simulink model "Block Diagram"  (R2024b)
settings: Solver=VariableStepAuto  StartTime=0.0  StopTime=10.0  RelTol=1e-3
libraries: simulink_extras x43, eeGeneralControl x4
(part 3 of 3)

== system Block Diagram/ALU/9-bit RCA/9bitRCA/1bitFAC2 ==
  y : Inport
  x : Inport  Port=2
  cin : Inport  Port=3
  AND : Logic  IconShape=distinctive  AllPortsSameDT=off  OutDataTypeStr=boolean
  AND1 : Logic  IconShape=distinctive  AllPortsSameDT=off  OutDataTypeStr=boolean
  AND2 : Logic  IconShape=distinctive  AllPortsSameDT=off  OutDataTypeStr=boolean
  OR : Logic  Operator=OR  Inputs=3  IconShape=distinctive  AllPortsSameDT=off  OutDataTypeStr=boolean
  XOR : Logic  Operator=XOR  Inputs=3  IconShape=distinctive  AllPortsSameDT=off  OutDataTypeStr=boolean
  z : Outport
  cout : Outport  Port=2
  wires:
  y/1 -> AND2/1, AND/2, XOR/2
  x/1 -> AND1/1, AND/1, XOR/1
  cin/1 -> AND2/2, AND1/2, XOR/3
  XOR/1 -> z/1
  OR/1 -> cout/1
  AND/1 -> OR/1
  AND1/1 -> OR/2
  AND2/1 -> OR/3

== system Block Diagram/ALU/9-bit RCA/9bitRCA/1bitFAC3 ==
  y : Inport
  x : Inport  Port=2
  cin : Inport  Port=3
  AND : Logic  IconShape=distinctive  AllPortsSameDT=off  OutDataTypeStr=boolean
  AND1 : Logic  IconShape=distinctive  AllPortsSameDT=off  OutDataTypeStr=boolean
  AND2 : Logic  IconShape=distinctive  AllPortsSameDT=off  OutDataTypeStr=boolean
  OR : Logic  Operator=OR  Inputs=3  IconShape=distinctive  AllPortsSameDT=off  OutDataTypeStr=boolean
  XOR : Logic  Operator=XOR  Inputs=3  IconShape=distinctive  AllPortsSameDT=off  OutDataTypeStr=boolean
  z : Outport
  cout : Outport  Port=2
  wires:
  y/1 -> AND2/1, AND/2, XOR/2
  x/1 -> AND1/1, AND/1, XOR/1
  cin/1 -> AND2/2, AND1/2, XOR/3
  XOR/1 -> z/1
  OR/1 -> cout/1
  AND/1 -> OR/1
  AND1/1 -> OR/2
  AND2/1 -> OR/3

== system Block Diagram/ALU/9-bit RCA/9bitRCA/1bitFAC4 ==
  y : Inport
  x : Inport  Port=2
  cin : Inport  Port=3
  AND : Logic  IconShape=distinctive  AllPortsSameDT=off  OutDataTypeStr=boolean
  AND1 : Logic  IconShape=distinctive  AllPortsSameDT=off  OutDataTypeStr=boolean
  AND2 : Logic  IconShape=distinctive  AllPortsSameDT=off  OutDataTypeStr=boolean
  OR : Logic  Operator=OR  Inputs=3  IconShape=distinctive  AllPortsSameDT=off  OutDataTypeStr=boolean
  XOR : Logic  Operator=XOR  Inputs=3  IconShape=distinctive  AllPortsSameDT=off  OutDataTypeStr=boolean
  z : Outport
  cout : Outport  Port=2
  wires:
  y/1 -> AND2/1, AND/2, XOR/2
  x/1 -> AND1/1, AND/1, XOR/1
  cin/1 -> AND2/2, AND1/2, XOR/3
  XOR/1 -> z/1
  OR/1 -> cout/1
  AND/1 -> OR/1
  AND1/1 -> OR/2
  AND2/1 -> OR/3

== system Block Diagram/ALU/9-bit RCA/9bitRCA/1bitFAC5 ==
  y : Inport
  x : Inport  Port=2
  cin : Inport  Port=3
  AND : Logic  IconShape=distinctive  AllPortsSameDT=off  OutDataTypeStr=boolean
  AND1 : Logic  IconShape=distinctive  AllPortsSameDT=off  OutDataTypeStr=boolean
  AND2 : Logic  IconShape=distinctive  AllPortsSameDT=off  OutDataTypeStr=boolean
  OR : Logic  Operator=OR  Inputs=3  IconShape=distinctive  AllPortsSameDT=off  OutDataTypeStr=boolean
  XOR : Logic  Operator=XOR  Inputs=3  IconShape=distinctive  AllPortsSameDT=off  OutDataTypeStr=boolean
  z : Outport
  cout : Outport  Port=2
  wires:
  y/1 -> AND2/1, AND/2, XOR/2
  x/1 -> AND1/1, AND/1, XOR/1
  cin/1 -> AND2/2, AND1/2, XOR/3
  XOR/1 -> z/1
  OR/1 -> cout/1
  AND/1 -> OR/1
  AND1/1 -> OR/2
  AND2/1 -> OR/3

== system Block Diagram/ALU/9-bit RCA/9bitRCA/1bitFAC6 ==
  y : Inport
  x : Inport  Port=2
  cin : Inport  Port=3
  AND : Logic  IconShape=distinctive  AllPortsSameDT=off  OutDataTypeStr=boolean
  AND1 : Logic  IconShape=distinctive  AllPortsSameDT=off  OutDataTypeStr=boolean
  AND2 : Logic  IconShape=distinctive  AllPortsSameDT=off  OutDataTypeStr=boolean
  OR : Logic  Operator=OR  Inputs=3  IconShape=distinctive  AllPortsSameDT=off  OutDataTypeStr=boolean
  XOR : Logic  Operator=XOR  Inputs=3  IconShape=distinctive  AllPortsSameDT=off  OutDataTypeStr=boolean
  z : Outport
  cout : Outport  Port=2
  wires:
  y/1 -> AND2/1, AND/2, XOR/2
  x/1 -> AND1/1, AND/1, XOR/1
  cin/1 -> AND2/2, AND1/2, XOR/3
  XOR/1 -> z/1
  OR/1 -> cout/1
  AND/1 -> OR/1
  AND1/1 -> OR/2
  AND2/1 -> OR/3

== system Block Diagram/ALU/9-bit RCA/9bitRCA/1bitFAC7 ==
  y : Inport
  x : Inport  Port=2
  cin : Inport  Port=3
  AND : Logic  IconShape=distinctive  AllPortsSameDT=off  OutDataTypeStr=boolean
  AND1 : Logic  IconShape=distinctive  AllPortsSameDT=off  OutDataTypeStr=boolean
  AND2 : Logic  IconShape=distinctive  AllPortsSameDT=off  OutDataTypeStr=boolean
  OR : Logic  Operator=OR  Inputs=3  IconShape=distinctive  AllPortsSameDT=off  OutDataTypeStr=boolean
  XOR : Logic  Operator=XOR  Inputs=3  IconShape=distinctive  AllPortsSameDT=off  OutDataTypeStr=boolean
  z : Outport
  cout : Outport  Port=2
  wires:
  y/1 -> AND2/1, AND/2, XOR/2
  x/1 -> AND1/1, AND/1, XOR/1
  cin/1 -> AND2/2, AND1/2, XOR/3
  XOR/1 -> z/1
  OR/1 -> cout/1
  AND/1 -> OR/1
  AND1/1 -> OR/2
  AND2/1 -> OR/3

== system Block Diagram/ALU/9-bit RCA/9bitRCA/1bitFAC8 ==
  y : Inport
  x : Inport  Port=2
  cin : Inport  Port=3
  AND : Logic  IconShape=distinctive  AllPortsSameDT=off  OutDataTypeStr=boolean
  AND1 : Logic  IconShape=distinctive  AllPortsSameDT=off  OutDataTypeStr=boolean
  AND2 : Logic  IconShape=distinctive  AllPortsSameDT=off  OutDataTypeStr=boolean
  OR : Logic  Operator=OR  Inputs=3  IconShape=distinctive  AllPortsSameDT=off  OutDataTypeStr=boolean
  XOR : Logic  Operator=XOR  Inputs=3  IconShape=distinctive  AllPortsSameDT=off  OutDataTypeStr=boolean
  z : Outport
  cout : Outport  Port=2
  wires:
  y/1 -> AND2/1, AND/2, XOR/2
  x/1 -> AND1/1, AND/1, XOR/1
  cin/1 -> AND2/2, AND1/2, XOR/3
  XOR/1 -> z/1
  OR/1 -> cout/1
  AND/1 -> OR/1
  AND1/1 -> OR/2
  AND2/1 -> OR/3

== system Block Diagram/ALU/Control Unit/modulo-3 phase counter/2-3 decoder ==
  d1 : Inport
  d0 : Inport  Port=2
  AND : Logic  IconShape=distinctive  AllPortsSameDT=off  OutDataTypeStr=boolean
  AND1 : Logic  IconShape=distinctive  AllPortsSameDT=off  OutDataTypeStr=boolean
  AND2 : Logic  IconShape=distinctive  AllPortsSameDT=off  OutDataTypeStr=boolean
  NOR : Logic  Operator=NOR  IconShape=distinctive  AllPortsSameDT=off  OutDataTypeStr=boolean
  NOT : Logic  Operator=NOT  IconShape=distinctive  AllPortsSameDT=off  OutDataTypeStr=boolean
  NOT1 : Logic  Operator=NOT  IconShape=distinctive  AllPortsSameDT=off  OutDataTypeStr=boolean
  Ph3 : Outport
  Ph2 : Outport  Port=2
  Ph1 : Outport  Port=3
  Ph0 : Outport  Port=4
  wires:
  d0/1 -> AND/2, NOR/2, NOT1/1, AND2/2
  d1/1 -> NOR/1, NOT/1, AND1/1, AND/1
  AND/1 -> Ph3/1
  NOR/1 -> Ph0/1
  AND1/1 -> Ph2/1
  AND2/1 -> Ph1/1
  NOT1/1 -> AND1/2
  NOT/1 -> AND2/1

== system Block Diagram/ALU/Control Unit/modulo-3 phase counter/modulo-3 counter ==
  clk : Inport
  rst : Inport  Port=2
  D Flip-Flop : simulink_extras/Flip Flops/D Flip-Flop
  D Flip-Flop1 : simulink_extras/Flip Flops/D Flip-Flop
  NOT : Logic  Operator=NOT  IconShape=distinctive  AllPortsSameDT=off  OutDataTypeStr=boolean
  b1 : Outport
  b0 : Outport  Port=2
  wires:
  clk/1 -> D Flip-Flop/2
  D Flip-Flop/2 -> b0/1, D Flip-Flop/1, D Flip-Flop1/2
  D Flip-Flop1/2 -> b1/1, D Flip-Flop1/1
  rst/1 -> NOT/1
  NOT/1 -> D Flip-Flop/3, D Flip-Flop1/3
